simulink model "ECE453_BlowerHw8"  (R2025a)
settings: Solver=VariableStepAuto  StartTime=0.0  StopTime=1.0  RelTol=1e-3
libraries: spsSeriesRLCBranchLib x5, spsCurrentMeasurementLib x2, spsDCVoltageSourceLib x2, spsVoltageMeasurementLib x2, spsDiodeLib x1, spsIdealSwitchLib x1, simulink x1, sps_lib x1
settings Model: Creator=cruisemac  LastModifiedBy=cruisemac

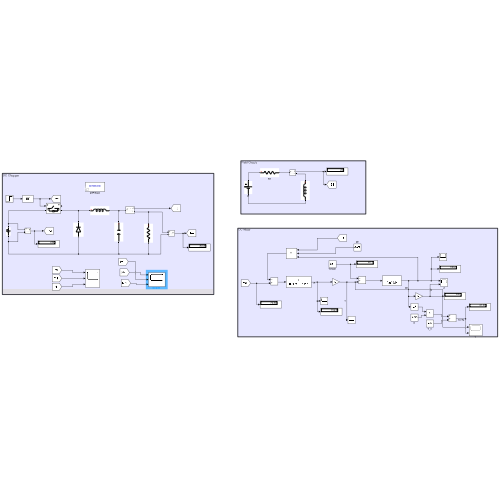
[thumbnail: Simulink's stored preview of the top-level diagram]
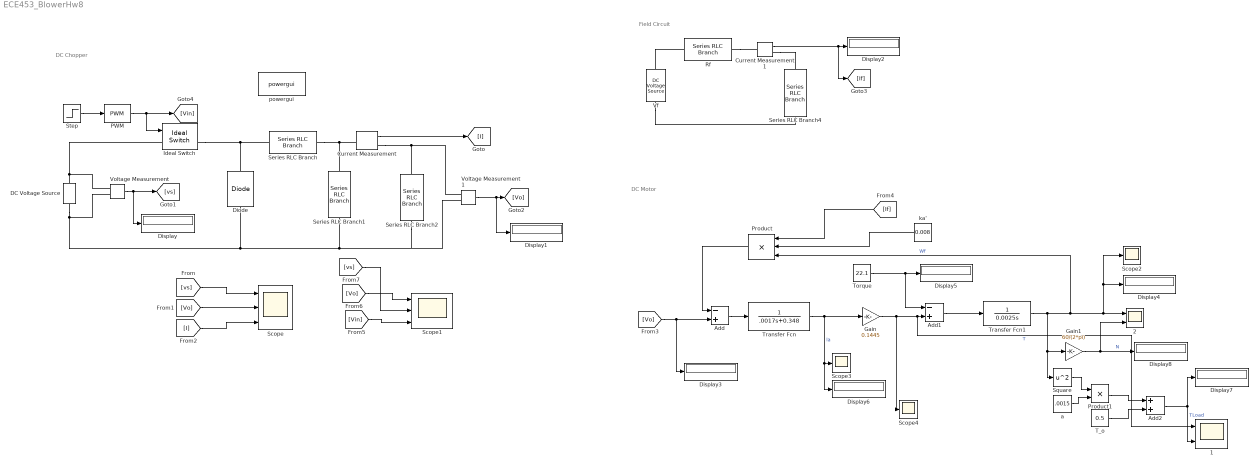
== system ECE453_BlowerHw8 ==
  note: DC Motor
  note: Field Circuit
  note: DC Chopper
  1 : Scope  NumInputPorts=2
      settings: ActiveDisplayYMinimum=-1  ActiveDisplayYMaximum=1  DataLoggingVariableName=ScopeData5
  2 : Scope  NumInputPorts=2
      settings: ActiveDisplayYMinimum=-821.95454482029368  ActiveDisplayYMaximum=2269.5930272142732
  Add : Sum  Inputs=-+
  Add1 : Sum  Inputs=-+
  Add2 : Sum
  Current Measurement : spsCurrentMeasurementLib/Current Measurement  PhasorSimulation=off  OutputType=Complex  PSBequivalent=0
  Current Measurement1 : spsCurrentMeasurementLib/Current Measurement  PhasorSimulation=off  OutputType=Complex  PSBequivalent=0
  DC Voltage Source : spsDCVoltageSourceLib/DC Voltage Source  Amplitude=260  Measurements=None
  Diode : spsDiodeLib/Diode  Ron=0.001  Lon=0  Vf=0.8  IC=0  UseSnubber=0  Rs=500  Cs=0  Measurements=off
  Display{,1..8} (9 alike) : Display
  Gain : Gain  Gain=0.1445
  Gain1 : Gain  Gain=60/(2*pi)
  Ideal Switch : spsIdealSwitchLib/Ideal Switch  Ron=0.001  Lon=0  IC=0  Rs=1e5  Cs=inf  Measurements=on
  PWM : simulink/Discontinuities/PWM  DisableCoverage=on  Period=.00005  InitialDelay=0  DisallowZeroDutyCycle=off  RunAtFixedTimeIntervals=off  SampleTime=0.1
  Product : Product  Inputs=3
  Product1 : Product
  Rf : spsSeriesRLCBranchLib/Series RLC Branch  LConnTagsString=__new0  RConnTagsString=__new0  BranchType=R  Resistance=0.5  Inductance=1e-3  SetiL0=off  InitialCurrent=0  Capacitance=1e-6  Setx0=off  InitialVoltage=0  Measurements=None
  Scope : Scope  NumInputPorts=3
      settings: ActiveDisplayYMinimum=60.707036751640928  ActiveDisplayYMaximum=91.47042738215292
  Scope1 : Scope  NumInputPorts=3
      settings: ActiveDisplayYMinimum=-41.23175275726652  ActiveDisplayYMaximum=301.48893049816093  DataLoggingVariableName=ScopeData6
  Scope2 : Scope
      settings: ActiveDisplayYMinimum=-408.70295414380951  ActiveDisplayYMaximum=1877.9930602583443  DataLoggingVariableName=ScopeData2
  Scope3 : Scope
      settings: ActiveDisplayYMinimum=-133.89077631166231  ActiveDisplayYMaximum=734.96856030372578  DataLoggingVariableName=ScopeData3
  Scope4 : Scope
      settings: ActiveDisplayYMinimum=-13.964538225488791  ActiveDisplayYMaximum=111.58563591543478  DataLoggingVariableName=ScopeData4
  Series RLC Branch : spsSeriesRLCBranchLib/Series RLC Branch  LConnTagsString=__new0  RConnTagsString=__new0  BranchType=L  Resistance=1  Inductance=180e-6  SetiL0=off  InitialCurrent=0  Capacitance=1e-6  Setx0=off  InitialVoltage=0  Measurements=None
  Series RLC Branch1 : spsSeriesRLCBranchLib/Series RLC Branch  LConnTagsString=__new0  RConnTagsString=__new0  BranchType=C  Resistance=1  Inductance=1e-3  SetiL0=off  InitialCurrent=0  Capacitance=100e-6  Setx0=off  InitialVoltage=0  Measurements=None
  Series RLC Branch2 : spsSeriesRLCBranchLib/Series RLC Branch  LConnTagsString=__new0  RConnTagsString=__new0  BranchType=R  Resistance=1  Inductance=1e-3  SetiL0=off  InitialCurrent=0  Capacitance=1e-6  Setx0=off  InitialVoltage=0  Measurements=None
  Series RLC Branch4 : spsSeriesRLCBranchLib/Series RLC Branch  LConnTagsString=__new0  RConnTagsString=__new0  BranchType=L  Resistance=1  Inductance=2e-3  SetiL0=off  InitialCurrent=0  Capacitance=1e-6  Setx0=off  InitialVoltage=0  Measurements=None
  Square : Math  Operator=square
  Step : Step  Time=0.6  Before=0.2805  After=0.30855  SampleTime=0
  T_o : Constant  Value=0.5
  Torque : Constant  Value=22.1
  Transfer Fcn : TransferFcn  Denominator=[.0017 0.348]
  Transfer Fcn1 : TransferFcn  Denominator=[0.0025 0]
  Vf : spsDCVoltageSourceLib/DC Voltage Source  Amplitude=10  Measurements=None
  Voltage Measurement : spsVoltageMeasurementLib/Voltage Measurement  PhasorSimulation=off  OutputType=Complex  PSBequivalent=0
  Voltage Measurement1 : spsVoltageMeasurementLib/Voltage Measurement  PhasorSimulation=off  OutputType=Complex  PSBequivalent=0
  a : Constant  Value=.0015
  ka' : Constant  Value=0.008
  powergui : sps_lib/powergui  Priority=1  SimulationMode=Continuous  SampleTime=50e-6  frequency=60  Iterations=50  frequencyindice=0  Pbase=100e6  ErrMax=1e-4  UnitsV=kV  UnitsW=MW  buscounter=0  FunctionMessages=off  echomessages=off  EnableUseOfTLC=off  CurrentSourceSwitches=off  DisableSnubberDevices=off  DisableRonSwitches=off  DisableVfSwitches=off  DisplayEquations=off  AutomaticDiscreteSolvers=off  SolverType=Tustin/Backward Euler (TBE)  Interpol=off  ExternalGateDelay=off  methode=off  Ts=100  x0status=blocks  SPID=on  SwTol=0  HookPort=off  NonlinearTolerance=1e-4  nMaxIteration=100  ContinueOnMaxIteration=off  RestoreLinks=warning  ResistiveCurrentMeasurement=off  Frange=[0:2:500]  Ylog=off  Xlog=on  ShowGrid=off  save=off  variable=ZData  structure=0  ZoomFFT=off  StartTime=0.0  cycles=1  DisplayStyle=1  fundamental=60  FreqAxis=off  MaxFrequency=1000  frequencyindicesteady=1  RmsSteady=1  display=off
  wires:
  [vs] -> Scope/1
  Voltage Measurement1/1 -> Display1/1, [Vo]
  [I] -> Scope/3
  Current Measurement/1 -> [I]
  Voltage Measurement/1 -> [vs], Display/1
  [Vo] -> Scope/2
  Current Measurement1/1 -> [If], Display2/1
  Transfer Fcn1/1 -> Product/3, Display4/1, Scope2/1, 2/1, Square/1, Gain1/1  "Wf"
  Product/1 -> Add/1
  Torque/1 -> Add1/1, Display5/1
  Add1/1 -> Transfer Fcn1/1
  Transfer Fcn/1 -> Display6/1, Scope3/1, Gain/1  "la"
  Gain/1 -> Scope4/1, 1/1, Add1/2  "T"
  ka'/1 -> Product/2
  Add/1 -> Transfer Fcn/1
  Gain1/1 -> Display8/1, 2/2  "N"
  [Vo] -> Display3/1, Add/2
  [If] -> Product/1
  PWM/1 -> [Vin], Ideal Switch/1
  Step/1 -> PWM/1
  a/1 -> Product1/2
  Square/1 -> Product1/1
  T_o/1 -> Add2/2
  Product1/1 -> Add2/1
  Add2/1 -> 1/2, Display7/1  "TLoad"
  [Vo] -> Scope1/1
  [Vin] -> Scope1/3
  [vs] -> Scope1/2
  connections:
  DC Voltage Source/LConn1 -- Voltage Measurement/LConn2 -- Diode/LConn1 -- Series RLC Branch2/RConn1 -- Voltage Measurement1/LConn2 -- Series RLC Branch1/RConn1
  Series RLC Branch/RConn1 -- Series RLC Branch1/LConn1 -- Current Measurement/LConn1
  Current Measurement/RConn1 -- Series RLC Branch2/LConn1 -- Voltage Measurement1/LConn1
  Ideal Switch/RConn1 -- Series RLC Branch/LConn1 -- Diode/RConn1
  Ideal Switch/LConn1 -- Voltage Measurement/LConn1 -- DC Voltage Source/RConn1
  Current Measurement1/RConn1 -- Series RLC Branch4/LConn1
  Vf/LConn1 -- Series RLC Branch4/RConn1
  Rf/RConn1 -- Current Measurement1/LConn1
  Vf/RConn1 -- Rf/LConn1
